simulink model "test_ale"  (R2026a)
settings: Solver=FixedStepAuto  StopTime=20
undefined symbols (not defined in the file): L, ld, psi_o, X_o, xRef, Y_o, yRef
libraries: robotalgslib x1, autolibshared x1
settings Model: SimulationMode=accelerator  Creator=Utente  LastModifiedBy=Utente

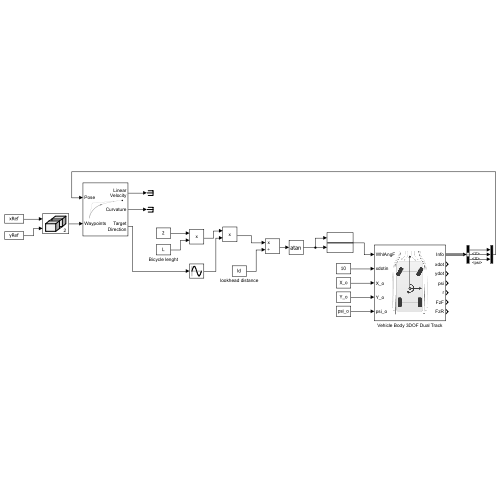
[thumbnail: Simulink's stored preview of the top-level diagram]
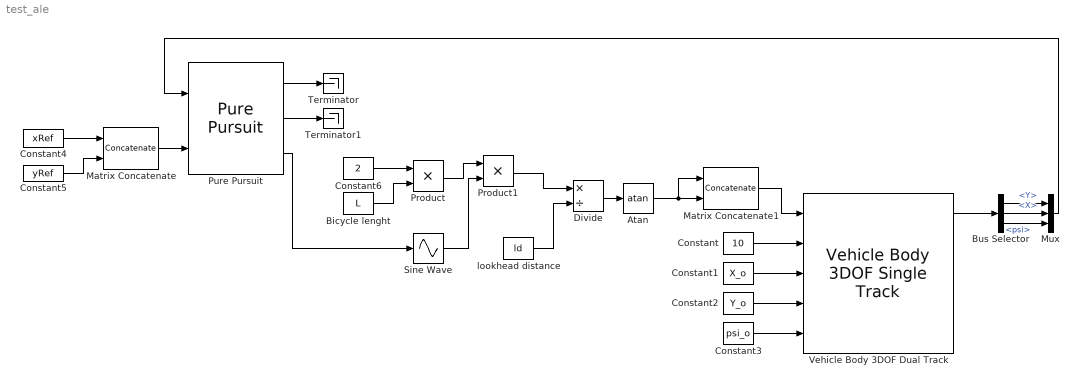
== system test_ale ==
  Atan : Trigonometry  Operator=atan
  Bicycle lenght : Constant  Value=L
  Bus Selector : BusSelector  OutputSignals=InertFrm.Cg.Disp.Y,InertFrm.Cg.Disp.X,InertFrm.Cg.Ang.psi
  Constant : Constant  Value=10
  Constant1 : Constant  Value=X_o
  Constant2 : Constant  Value=Y_o
  Constant3 : Constant  Value=psi_o
  Constant4 : Constant  Value=xRef
  Constant5 : Constant  Value=yRef
  Constant6 : Constant  Value=2
  Divide : Product  Inputs=*/
  Matrix Concatenate : Concatenate  Mode=Multidimensional array  ConcatenateDimension=2
  Matrix Concatenate1 : Concatenate  ConcatenateDimension=2
  Mux : Mux  Inputs=3
  Product : Product
  Product1 : Product
  Pure Pursuit : robotalgslib/Pure Pursuit  DesiredLinearVelocityPort=off  DesiredLinearVelocity=0.1  MaxCurvature=1.0  LookaheadDistancePort=off  LookaheadDistance=ld  TargetDirPort=on  SimulateUsing=Code generation
      settings: LibrarySourceBlock=robotmobilelib/Pure Pursuit
  Sine Wave : Sin  TimeSource=Use external signal  SampleTime=0
  Terminator : Terminator
  Terminator1 : Terminator
  Vehicle Body 3DOF Dual Track : autolibshared/Vehicle Body 3DOF Single Track  trackMode=Dual  inputMode=External longitudinal velocity  frontSteerMode=on  rearSteerMode=off  extFMode=off  htchFMode=off  extMMode=off  htchMMode=off  windMode=off  extTamb=off  muMode=off  extGndPlnElev=off  extGndPlnRoll=off  extGndPlnPitch=off  extGndPlnDCM=off  extXo=on  extxdoto=off  extYo=on  extydoto=off  extpsio=on  extro=off  aMode=2  NF=2  NR=2  m=2000  a=1.4  b=1.6  h=0.35  dh=1  hh=0.2  X_o=0  xdot_o=0  d=0  hl=0  w=[1.4,1.4]  CalphaMode=Constant  sigmaMode=on  sigma_f=.1  sigma_r=.1  Cy_f=12e3  Cy_r=11e3  Cy_f_data="[1.396121365092108e+04\t4.232462640127975e+04\t6.754894575573687e+04\t8.835784428391886e+04\t1.043551700699839e+05\t1.158335754468729e+05\t1.234691551560788e+05\t1.280575366661118e+05\t1.298126639907242e+05\t1.298126639907242e+05]"  alpha_f_brk=[-0.785, -0.628, -0.471, -0.314, -0.157, 0.000, 0.157, 0.314, 0.471, 0.628, 0.785]  Fz_f_brk="[500\t1.555555555555556e+03\t2.611111111111111e+03\t3.666666666666667e+03\t4.722222222222223e+03\t5.777777777777777e+03\t6.833333333333333e+03\t7.888888888888889e+03\t8.944444444444445e+03\t10000]"  Cy_r_data="[1.396121365092108e+04\t4.232462640127975e+04\t6.754894575573687e+04\t8.835784428391886e+04\t1.043551700699839e+05\t1.158335754468729e+05\t1.234691551560788e+05\t1.280575366661118e+05\t1.298126639907242e+05\t1.298126639907242e+05]"  alpha_r_brk=[-0.785, -0.628, -0.471, -0.314, -0.157, 0.000, 0.157, 0.314, 0.471, 0.628, 0.785]  Fz_r_brk="[500\t1.555555555555556e+03\t2.611111111111111e+03\t3.666666666666667e+03\t4.722222222222223e+03\t5.777777777777777e+03\t6.833333333333333e+03\t7.888888888888889e+03\t8.944444444444445e+03\t10000]"  Fznom=5000  Y_o=0  ydot_o=0  Izz=4000  psi_o=0  r_o=0  Af=2  Cd=.3  Cl=.1  Cpm=.1  beta_w=[0 0.01:0.01:0.3]  Cs=[0:0.03:0.9]  Cym=[0 1e-6:0.01:0.3]  Pabs=101325  Tair=273  g=9.81  mu=1  GndPlnRoll=0  GndPlnPitch=0  GndPlnElev=0  xdot_tol=.01  Fxtire_sat=7e4  Fytire_sat=7e4  longOff=0  latOff=0  vertOff=0.35  wrapAng=off
      settings: LibrarySourceBlock=vehdynlibeom/Vehicle Body 3DOF Dual Track
  lookhead distance : Constant  Value=ld
  wires:
  Constant/1 -> Vehicle Body 3DOF Dual Track/2
  Constant1/1 -> Vehicle Body 3DOF Dual Track/3
  Constant2/1 -> Vehicle Body 3DOF Dual Track/4
  Constant3/1 -> Vehicle Body 3DOF Dual Track/5
  Constant4/1 -> Matrix Concatenate/1
  Constant5/1 -> Matrix Concatenate/2
  Matrix Concatenate/1 -> Pure Pursuit/2
  Vehicle Body 3DOF Dual Track/1 -> Bus Selector/1
  Bus Selector/1 -> Mux/1  "<Y>"
  Bus Selector/3 -> Mux/3  "<psi>"
  Bus Selector/2 -> Mux/2  "<X>"
  Mux/1 -> Pure Pursuit/1
  Constant6/1 -> Product/1
  Bicycle lenght/1 -> Product/2
  Product1/1 -> Divide/1
  lookhead distance/1 -> Divide/2
  Atan/1 -> Matrix Concatenate1/2, Matrix Concatenate1/1
  Divide/1 -> Atan/1
  Product/1 -> Product1/1
  Sine Wave/1 -> Product1/2
  Pure Pursuit/3 -> Sine Wave/1
  Matrix Concatenate1/1 -> Vehicle Body 3DOF Dual Track/1
  Pure Pursuit/1 -> Terminator/1
  Pure Pursuit/2 -> Terminator1/1
